simulink model "VLC"  (R2018b)
settings: Solver=FixedStepDiscrete  StartTime=0.0  StopTime=inf  FixedStep=0.01  RelTol=1e-3
PostLoadFcn:
  | if any(exist('dsrtsu_mdlpostloadfcn', 'file') ~= 0), dsrtsu_mdlpostloadfcn('Execute', bdroot); end
values from neighbouring files (symbols this model uses):
  m_Vehicle = 2000.0    [VLC_Local.sldd]
  P_A = 2.0    [VLC_Local.sldd]
  P_aDiffaF = 0.05    [VLC_Local.sldd]
  P_Cd = 0.29    [VLC_Local.sldd]
  P_Cf = 0.1    [VLC_Local.sldd]
  P_dAxMax = 2.0    [VLC_Local.sldd]
  P_dAxMin = -4.0    [VLC_Local.sldd]
  P_DC2ECMargin = 0.1    [VLC_Local.sldd]
  P_Dev4IEnd = 0.1    [VLC_Local.sldd]
  P_dIRamp = 1.0    [VLC_Local.sldd]
  P_DriveOffAdd = 400.0    [VLC_Local.sldd]
  P_dSlopeLim = 0.3    [VLC_Local.sldd]
  P_Ki = 0.08    [VLC_Local.sldd]
  P_Kp = 0.2    [VLC_Local.sldd]
  P_SlopeMax = 2.0    [VLC_Local.sldd]
  P_SlopeMin = 0.2    [VLC_Local.sldd]
  P_StandStillFactEC = 1.0    [VLC_Local.sldd]
  P_StsdCase = 1.0    [VLC_Local.sldd]
  P_StsddAxRamp = 1.0    [VLC_Local.sldd]
  P_tARefFilter = 0.2    [VLC_Local.sldd]
  P_tDriveOffThr = 5.0    [VLC_Local.sldd]
  P_tFxMergeFilter = 0.1    [VLC_Local.sldd]
  P_tSlopeFilter1 = 0.4    [VLC_Local.sldd]
  P_tSlopeFilter2 = 0.1    [VLC_Local.sldd]
  P_vDriveOffThr = 1.4    [VLC_Local.sldd]
  P_vLowSpd = 0.83    [VLC_Local.sldd]
  r_Wheel = 0.347    [VLC_Local.sldd]
  TransRatio = 7.38    [VLC_Local.sldd]
libraries: LPFilter x4
settings Model: DSRTSU_INTERNAL_RTI_VER=540  DSRTSU_INTERNAL_RTI_TYPE=rti1401  RTICANMMDATA=struct('GeneralSetupData',struct('modelroot','F:\DatabaseZO\08.Code\Model\ZOP_Integration','generalsettings',struct('filesettings',struct('destfolder',struct('Name','RTICANMM_FILES','Check',1),'buildfolder',struct('Name','.','Check',1),'AbsDestfolder',struct('Name','F:\DatabaseZO\08.Code\Model\ZOP_Integration\RTICANMM_FILES'),'AbsBuildfolder',struct('Name','F:\DatabaseZO\08.Code\Model\ZOP_Integration'))),'options',struct('addpaths',1,'rmpaths',1,'addtrcexclusion',logical(1),'cannavigator',struct('checkmonitoring',0),'show_usrtrc',0,'use_usrtrc',0),'advanced',struct('options',ones(1,100)),'MPSetup',{{}},'RTI',struct('Type','RTI1401','Ver','7.12','Date','02-May-2019'),'modelname','VLC','block','VLC'))  DSRTSU_INTERNAL_RTIFPGA=130  Creator=Administrator  LastModifiedBy=zjw
settings OptimizationCC: BlockReduction=off  ConditionallyExecuteInputs=off  OptimizeBlockIOStorage=off  BufferReuse=off  GlobalBufferReuse=off  ExpressionFolding=off  PassReuseOutputArgsThreshold=0  LocalBlockOutputs=off  OptimizeBlockOrder=speed  OptimizeDataStoreBuffers=off  BusAssignmentInplaceUpdate=off
settings DebuggingCC: ParameterTunabilityLossMsg=error  BusObjectLabelMismatch=none
settings HardwareCC: ProdBitPerPointer=32  ProdBitPerSizeT=32  ProdBitPerPtrDiffT=32  ProdLargestAtomicInteger=Integer  ProdEndianess=BigEndian  ProdWordSize=32  ProdHWDeviceType=Custom Processor->Custom  TargetIntDivRoundTo=Zero  TargetEndianess=BigEndian  TargetHWDeviceType=Custom Processor->Custom
settings ModelReferenceCC: ModelReferenceNumInstancesAllowed=Single
settings SFSimCC: MATLABDynamicMemAlloc=off
settings RTWCC: SystemTargetFile=rti1401.tlc  MakeCommand=make_rti  TemplateMakefile=rti1401.tmf  Description=dSPACE DS1401 Hardware Platform  GenerateReport=on  LaunchReport=on
settings CodeAppCC: OperatorAnnotations=on
settings STFCustomTargetCC: ParMdlRefBuildCompliant=on  SystemTargetFile=rti1401.tlc
settings GRTTargetCC: TargetLangStandard=C89/C90 (ANSI)  CompOptLevelCompliant=off  ConcurrentExecutionCompliant=off  CombineOutputUpdateFcns=off  MatFileLogging=off  CPPClassGenCompliant=off  UseToolchainInfoCompliant=off

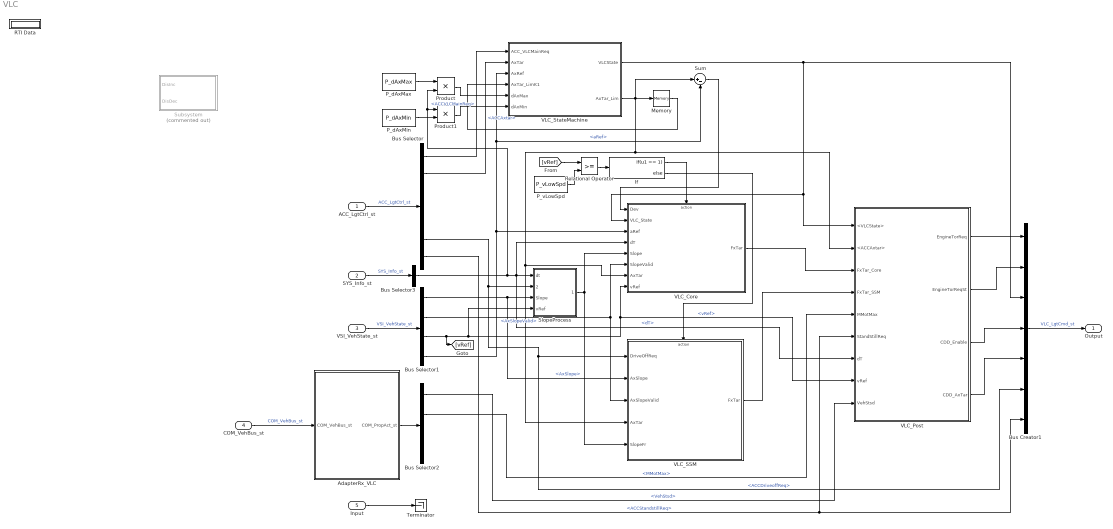
== system VLC ==
  ACC_LgtCtrl_st : Inport  OutDataTypeStr=Bus: ACC_LGTCTRL_ST  BusOutputAsStruct=on
  SYS_Info_st : Inport  Port=2  OutDataTypeStr=Bus: SYS_INFO_ST  BusOutputAsStruct=on
  VSI_VehState_st : Inport  Port=3  OutDataTypeStr=Bus: VSI_VEHSTATE_ST  BusOutputAsStruct=on
  COM_VehBus_st : Inport  Port=4  OutDataTypeStr=Bus: COM_VEHBUS_ST  BusOutputAsStruct=on
  Input : Inport  Port=5  OutDataTypeStr=Bus: COM_PROPACT_ST  BusOutputAsStruct=on
  AdapterRx_VLC : Subsystem
  Bus Creator1 : BusCreator  Inputs=7  OutDataTypeStr=Bus: VLC_LGTCMD_ST  NonVirtualBus=on
  Bus Selector : BusSelector  OutputSignals=ACCVLCMainReq,ACCAxtar,ACCAxTarUpperComfBand,ACCAxTarLowerComfBand,ACCBrkPrfrd,ACCDriveoffReq,ACCStandstillReq
  Bus Selector1 : BusSelector  OutputSignals=AxSlope,AxSlopeValid,vRef,aRef
  Bus Selector2 : BusSelector  OutputSignals=VehStsd,MMotMax,MMotMin,BrakeForce
  Bus Selector3 : BusSelector  OutputSignals=dT
  If : If  IfExpression=u1 == 1
  Memory : Memory
  P_dAxMax : Constant  Value=P_dAxMax
  P_dAxMin : Constant  Value=P_dAxMin
  P_vLowSpd : Constant  Value=P_vLowSpd
  Product : Product
  Product1 : Product
  RTI Data : Subsystem  Tag=struct('RTIDataServer',struct('RTIDataServerVs','2','RTIModelDescription','struct(''main'',''VLC'',''sub'','''',''isMp'',0)'))  LoadFcn="if exist('rtidc'), try,  rtidc('DataHostBlockClbLoad', gcbh); catch, disp(['Warning: ''LoadFcn'' for RTI Data block failed: ' lasterr]); end, end,"  mask(RTI_DATA_HOST){}
      mask help:
      | RTI Data Block.
      | This block is used by RTI to store internal model-dependent data.
      | Please keep this block on the root level of the model. Deleting this block will result in data loss.
      |
      | NEVER DELETE OR COPY THIS BLOCK!
      settings: CopyFcn="if exist('rtidc'), try,  rtidc('DataHostBlockClbCopy', gcbh); catch, disp(['Warning: ''CopyFcn'' for RTI Data block failed: ' lasterr]); end, end,"  DeleteFcn="if exist('rtidc'), try,  rtidc('DataHostBlockClbDelete', gcbh); catch, disp(['Warning: ''DeleteFcn'' for RTI Data block failed: ' lasterr]); end, end,"  ModelCloseFcn="if exist('rtidc'), try,  rtidc('DataHostBlockClbModelClose', gcbh); catch, disp(['Warning: ''ModelCloseFcn'' for RTI Data block failed: ' lasterr]); end, end,"  PreSaveFcn="if exist('rtidc'), try,  rtidc('DataHostBlockClbPreSave', gcbh); catch, disp(['Warning: ''PreSaveFcn'' for RTI Data block failed: ' lasterr]); end, end,"  PostSaveFcn="if exist('rtidc'), try,  rtidc('DataHostBlockClbPostSave', gcbh); catch, disp(['Warning: ''PostSaveFcn'' for RTI Data block failed: ' lasterr]); end, end,"  NameChangeFcn="if exist('rtidc'), try,  rtidc('DataHostBlockClbNameChange', gcbh); catch, disp(['Warning: ''NameChangeFcn'' for RTI Data block failed: ' lasterr]); end, end,"
      mask Help:
      | RTI Data Block.
      | This block is used by RTI to store internal model-dependent data.
      | Please keep this block on the root level of the model. Deleting this block will result in data loss.
      | 
      | NEVER DELETE OR COPY THIS BLOCK!
      mask Display:
      | text(0.5, 0.5, 'RTI Data', 'HorizontalAlignment', 'center');
      | plot([1 0]);
  Relational Operator : RelationalOperator  OutDataTypeStr=boolean  RndMeth=Simplest
  SlopeProcess : Subsystem
  Subsystem : Subsystem  Commented=on
  Sum : Sum  Inputs=|+-
  Terminator : Terminator
  VLC_Core : Subsystem
  VLC_Post : Subsystem
  VLC_SSM : Subsystem
  VLC_StateMachine : Stateflow chart  TreatAsAtomicUnit=on
  Output : Outport  OutDataTypeStr=Bus: VLC_LGTCMD_ST  BusOutputAsStruct=on
  wires:
  VSI_VehState_st/1 -> Bus Selector1/1  "VSI_VehState_st"
  If/1 -> VLC_Core/Action
  Bus Selector/2 -> VLC_StateMachine/2(AxTar)  "<ACCAxtar>"
  Bus Selector1/4 -> Sum/2, VLC_StateMachine/3(AxRef), VLC_Core/3(aRef)  "<aRef>"
  Bus Selector1/3 -> [vRef], SlopeProcess/4(vRef), VLC_Post/8(vRef), VLC_Core/8(vRef)  "<vRef>"
  If/2 -> VLC_SSM/Action
  Bus Selector/6 -> SlopeProcess/2(DriveOffReq), Bus Creator1/6, VLC_SSM/1(DriveOffReq)  "<ACCDriveoffReq>"
  Bus Selector1/2 -> VLC_SSM/3(AxSlopeValid), VLC_Core/6(SlopeValid)  "<AxSlopeValid>"
  Sum/1 -> VLC_Core/1(Dev)
  VLC_Core/1(FxTar) -> VLC_Post/3(FxTar_Core)
  VLC_SSM/1(FxTar) -> VLC_Post/4(FxTar_SSM)
  Bus Selector2/2 -> VLC_Post/5(MMotMax)  "<MMotMax>"
  Bus Selector/1 -> VLC_StateMachine/1(ACC_VLCMainReq)  "<ACCVLCMainReq>"
  VLC_StateMachine/1(VLCState) -> Bus Creator1/3, VLC_Post/1(<VLCState>), VLC_Core/2(VLC_State)
  VLC_StateMachine/2(AxTar_Lim) -> Memory/1, VLC_Post/2(<ACCAxtar>), VLC_SSM/4(AxTar), VLC_Core/7(AxTar), Sum/1
  Memory/1 -> VLC_StateMachine/4(AxTar_LimK1)
  VLC_Post/1(EngineTorReq) -> Bus Creator1/1
  VLC_Post/2(EngineTorReqSt) -> Bus Creator1/2
  VLC_Post/3(CDD_Enable) -> Bus Creator1/4
  VLC_Post/4(CDD_AxTar) -> Bus Creator1/5
  Bus Selector/7 -> Bus Creator1/7, VLC_Post/6(StandStillReq)  "<ACCStandstillReq>"
  SYS_Info_st/1 -> Bus Selector3/1  "SYS_Info_st"
  Bus Selector3/1 -> VLC_Post/7(dT), SlopeProcess/1(dt), VLC_Core/4(dT), Product/2, Product1/1  "<dT>"
  ACC_LgtCtrl_st/1 -> Bus Selector/1  "ACC_LgtCtrl_st"
  Product/1 -> VLC_StateMachine/5(dAxMax)
  P_dAxMax/1 -> Product/1
  AdapterRx_VLC/1(COM_PropAct_st) -> Bus Selector2/1
  COM_VehBus_st/1 -> AdapterRx_VLC/1(COM_VehBus_st)  "COM_VehBus_st"
  Bus Creator1/1 -> Output/1  "VLC_LgtCmd_st"
  Input/1 -> Terminator/1
  Bus Selector1/1 -> VLC_SSM/2(AxSlope), SlopeProcess/3(Slope)  "<AxSlope>"
  P_dAxMin/1 -> Product1/2
  Product1/1 -> VLC_StateMachine/6(dAxMin)
  SlopeProcess/1(SlopeFr) -> VLC_SSM/5(SlopeFr), VLC_Core/5(Slope)
  Bus Selector2/1 -> VLC_Post/9(VehStsd)  "<VehStsd>"
  P_vLowSpd/1 -> Relational Operator/2
  [vRef] -> Relational Operator/1
  Relational Operator/1 -> If/1

== system VLC/AdapterRx_VLC ==
  COM_VehBus_st : Inport  OutDataTypeStr=Bus: COM_VEHBUS_ST
  Bus Creator2 : BusCreator  Inputs=4  OutDataTypeStr=Bus: COM_PROPACT_ST  NonVirtualBus=on
  Bus Selector : BusSelector  OutputSignals=x251.VehSdslSts,xAC.EPTTrInptShaftMaxAvlblToq,xAC.EPTTrInptShaftMinAvlblToq,x24C.WhlBrkPrsSts
  Cast To Boolean : DataTypeConversion  OutDataTypeStr=single
  Divide : Product  Inputs=**
  Divide1 : Product  Inputs=**
  Logical Operator7 : Logic  Operator=NOT  AllPortsSameDT=off  OutDataTypeStr=boolean
  TransRatio : Constant  Value=TransRatio
  COM_PropAct_st : Outport  OutDataTypeStr=Bus: COM_PROPACT_ST
  wires:
  Bus Creator2/1 -> COM_PropAct_st/1  "COM_PropAct_st"
  Logical Operator7/1 -> Bus Creator2/4  "BrakeForce"
  Divide1/1 -> Bus Creator2/3  "MMotMin"
  Divide/1 -> Bus Creator2/2  "MMotMax"
  COM_VehBus_st/1 -> Bus Selector/1  "COM_VehBus_st"
  Bus Selector/4 -> Logical Operator7/1  "<WhlBrkPrsSts>"
  TransRatio/1 -> Divide/2, Divide1/2
  Bus Selector/2 -> Divide/1  "<EPTTrInptShaftMaxAvlblToq>"
  Bus Selector/3 -> Divide1/1  "<EPTTrInptShaftMinAvlblToq>"
  Bus Selector/1 -> Cast To Boolean/1  "<VehSdslSts>"
  Cast To Boolean/1 -> Bus Creator2/1  "VehStsd"

== system VLC/RTI Data ==
  RTI Data Store : Subsystem  Tag="struct('private',struct('version',struct('dsVer',uint32(2),'dsVerCreation',uint32(2),'RTI',struct('ver','7.12','type','RTI1401')),'access',struct('type','Model','isPerm',1,'created',['20-Nov-2020 12:07:07'],'modified',['07-Jan-2021 20:10:10'],'location','')),'public',struct('main',struct('data',[]),'sub',struct('name',{{'VLC'}},'data',{{struct('TH',struct('thTaskInfo',struct('taskType',{'TIMER','HWINT','TMRINT','SWINT','GLINT'},'tasksNumOf',{1,0,0,0,0},'srcIds',{{'TIMERA'},{},{},{},{}},'taskNames',{{['Timer Task 1']},{},{},{},{}})),'th_tc',struct('dataType','TASK','taskGroupId','','taskGroupList',{{}},'taskSchedulingPolicy','FCFS','taskType','TIMER','blkh',-1,'srcId','TIMERA','srcSgnName',['Timer A interrupt'],'srcCpuName','','taskName',['Timer Task 1  [0.01] s'],'taskNameDisplayExt','','smplTime',0.01,'smplTimeOffs',0,'hasFixedPriority',0,'priority',1,'hasFixedOvc',0,'ovcType',1,'ovcMax',1),'tc_th',struct('dataType','TASK','taskGroupId','','taskGroupList',{{}},'taskSchedulingPolicy','FCFS','taskType','TIMER','blkh',-1,'srcId','TIMERA','srcSgnName',['Timer A interrupt'],'srcCpuName','','taskName',['Timer Task 1  [0.01] s'],'taskNameDisplayExt','','smplTime',0.01,'smplTimeOffs',0,'hasFixedPriority',0,'priority',1,'hasFixedOvc',0,'ovcType',3,'ovcMax',1))}})))"  mask(RTI_DATA_STORE){}
      mask help:
      | RTI Data Store Block. This block is used by RTI to store internal model dependent data. Deleting this block will result in data loss.
      |
      | NEVER DELETE, COPY, OR MODIFY THIS BLOCK!
      mask Help:
      | RTI Data Store Block. This block is used by RTI to store internal model dependent data. Deleting this block will result in data loss.
      | 
      | NEVER DELETE, COPY, OR MODIFY THIS BLOCK!
      mask Display: text(0.5, 0.5, ' ', 'HorizontalAlignment', 'center');

== system VLC/SlopeProcess ==
  dt : Inport
  DriveOffReq : Inport  Port=2
  Slope : Inport  Port=3
  vRef : Inport  Port=4
  SlopeF : Subsystem
  SlopeFreeze : Subsystem
  SlopeFr : Outport
  wires:
  dt/1 -> SlopeFreeze/3(dT), SlopeF/1(dt)
  SlopeF/1(SlopeF) -> SlopeFreeze/4(SlopeF)
  SlopeFreeze/1(SlopeFreeze) -> SlopeFr/1
  Slope/1 -> SlopeF/2(Slope)
  vRef/1 -> SlopeFreeze/1(vVeh)
  DriveOffReq/1 -> SlopeFreeze/2(DriveOffReq)

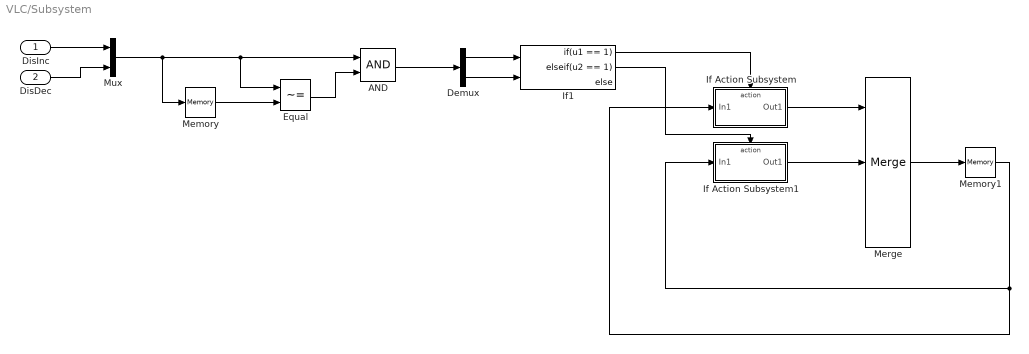
== system VLC/Subsystem ==
  DisInc : Inport
  DisDec : Inport  Port=2
  AND : Logic  AllPortsSameDT=off  OutDataTypeStr=boolean
  Demux : Demux  Outputs=2
  Equal : RelationalOperator  Operator=~=  OutDataTypeStr=boolean  RndMeth=Simplest
  If Action Subsystem : Subsystem  TreatAsAtomicUnit=on
  If Action Subsystem1 : Subsystem  TreatAsAtomicUnit=on
  If1 : If  NumInputs=2  IfExpression=u1 == 1  ElseIfExpressions=u2 == 1
  Memory : Memory
  Memory1 : Memory
  Merge : Merge  Inputs=3
  Mux : Mux  Inputs=2
  wires:
  Mux/1 -> Memory/1, Equal/1, AND/1
  Equal/1 -> AND/2
  Memory/1 -> Equal/2
  DisInc/1 -> Mux/1
  DisDec/1 -> Mux/2
  AND/1 -> Demux/1
  Demux/1 -> If1/1
  Demux/2 -> If1/2
  If1/1 -> If Action Subsystem/Action
  If Action Subsystem/1(Out1) -> Merge/1
  Merge/1 -> Memory1/1
  Memory1/1 -> If Action Subsystem1/1(In1), If Action Subsystem/1(In1)
  If Action Subsystem1/1(Out1) -> Merge/2
  If1/2 -> If Action Subsystem1/Action

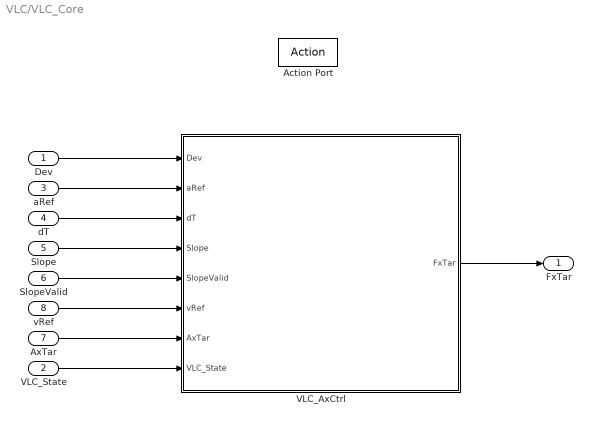
== system VLC/VLC_Core ==
  Dev : Inport
  VLC_State : Inport  Port=2
  aRef : Inport  Port=3
  dT : Inport  Port=4
  Slope : Inport  Port=5
  SlopeValid : Inport  Port=6
  AxTar : Inport  Port=7
  vRef : Inport  Port=8
  Action Port : ActionPort  ActionType=then
  VLC_AxCtrl : Subsystem
  FxTar : Outport
  wires:
  Dev/1 -> VLC_AxCtrl/1(Dev)
  VLC_AxCtrl/1(FxTar) -> FxTar/1
  aRef/1 -> VLC_AxCtrl/2(aRef)
  dT/1 -> VLC_AxCtrl/3(dT)
  Slope/1 -> VLC_AxCtrl/4(Slope)
  SlopeValid/1 -> VLC_AxCtrl/5(SlopeValid)
  vRef/1 -> VLC_AxCtrl/6(vRef)
  AxTar/1 -> VLC_AxCtrl/7(AxTar)
  VLC_State/1 -> VLC_AxCtrl/8(VLC_State)

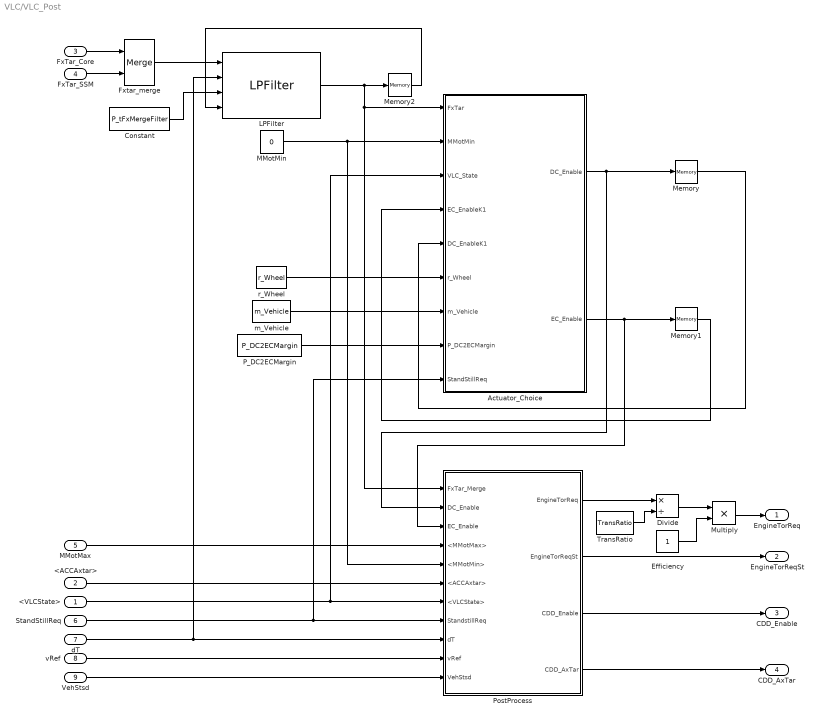
== system VLC/VLC_Post ==
  <VLCState> : Inport
  <ACCAxtar> : Inport  Port=2
  FxTar_Core : Inport  Port=3
  FxTar_SSM : Inport  Port=4
  MMotMax : Inport  Port=5
  StandStillReq : Inport  Port=6
  dT : Inport  Port=7
  vRef : Inport  Port=8
  VehStsd : Inport  Port=9
  Actuator_Choice : MATLAB Function  TreatAsAtomicUnit=on
  Constant : Constant  Value=P_tFxMergeFilter  OutDataTypeStr=single
  Divide : Product  Inputs=*/
  Efficiency : Constant
  Fxtar_merge : Merge
  LPFilter : LPFilter/LPFilter  SystemSampleTime=-1
      settings: SourceProductName=CustomLib
  MMotMin : Constant  Value=0  OutDataTypeStr=single
  Memory : Memory
  Memory1 : Memory
  Memory2 : Memory
  Multiply : Product  OutDataTypeStr=single
  P_DC2ECMargin : Constant  Value=P_DC2ECMargin
  PostProcess : Subsystem
  TransRatio : Constant  Value=TransRatio
  m_Vehicle : Constant  Value=m_Vehicle
  r_Wheel : Constant  Value=r_Wheel
  EngineTorReq : Outport
  EngineTorReqSt : Outport  Port=2
  CDD_Enable : Outport  Port=3
  CDD_AxTar : Outport  Port=4
  wires:
  MMotMin/1 -> Actuator_Choice/2(MMotMin), PostProcess/5(<MMotMin>)
  Actuator_Choice/1(DC_Enable) -> PostProcess/2(DC_Enable), Memory/1
  Memory/1 -> Actuator_Choice/5(DC_EnableK1)
  Actuator_Choice/2(EC_Enable) -> PostProcess/3(EC_Enable), Memory1/1
  Memory1/1 -> Actuator_Choice/4(EC_EnableK1)
  FxTar_SSM/1 -> Fxtar_merge/2
  FxTar_Core/1 -> Fxtar_merge/1
  MMotMax/1 -> PostProcess/4(<MMotMax>)
  <ACCAxtar>/1 -> PostProcess/6(<ACCAxtar>)
  <VLCState>/1 -> PostProcess/7(<VLCState>), Actuator_Choice/3(VLC_State)
  PostProcess/2(EngineTorReqSt) -> EngineTorReqSt/1
  PostProcess/3(CDD_Enable) -> CDD_Enable/1
  PostProcess/4(CDD_AxTar) -> CDD_AxTar/1
  r_Wheel/1 -> Actuator_Choice/6(r_Wheel)
  P_DC2ECMargin/1 -> Actuator_Choice/8(P_DC2ECMargin)
  m_Vehicle/1 -> Actuator_Choice/7(m_Vehicle)
  StandStillReq/1 -> PostProcess/8(StandstillReq), Actuator_Choice/9(StandStillReq)
  PostProcess/1(EngineTorReq) -> Divide/1
  TransRatio/1 -> Divide/2
  Divide/1 -> Multiply/1
  Multiply/1 -> EngineTorReq/1
  Efficiency/1 -> Multiply/2
  dT/1 -> PostProcess/9(dT), LPFilter/2
  LPFilter/1 -> Memory2/1, PostProcess/1(FxTar_Merge), Actuator_Choice/1(FxTar)
  Fxtar_merge/1 -> LPFilter/1
  Memory2/1 -> LPFilter/4
  Constant/1 -> LPFilter/3
  vRef/1 -> PostProcess/10(vRef)
  VehStsd/1 -> PostProcess/11(VehStsd)

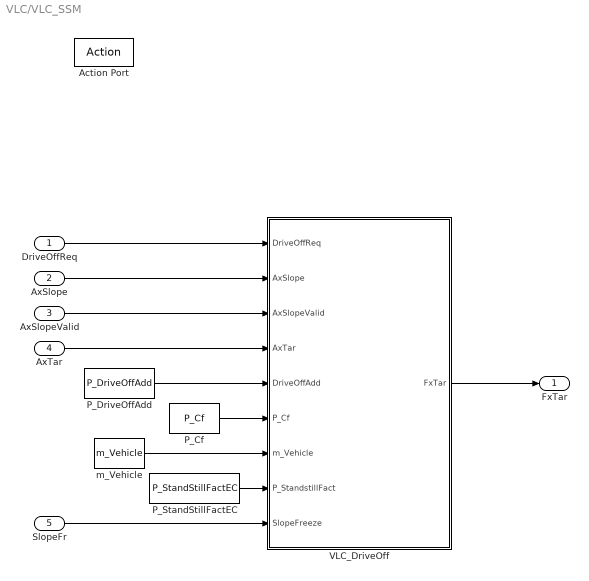
== system VLC/VLC_SSM ==
  DriveOffReq : Inport
  AxSlope : Inport  Port=2
  AxSlopeValid : Inport  Port=3
  AxTar : Inport  Port=4
  SlopeFr : Inport  Port=5
  Action Port : ActionPort  ActionType=else
  P_Cf : Constant  Value=P_Cf
  P_DriveOffAdd : Constant  Value=P_DriveOffAdd
  P_StandStillFactEC : Constant  Value=P_StandStillFactEC
  VLC_DriveOff : MATLAB Function  TreatAsAtomicUnit=on
  m_Vehicle : Constant  Value=m_Vehicle
  FxTar : Outport  OutDataTypeStr=single
  wires:
  DriveOffReq/1 -> VLC_DriveOff/1(DriveOffReq)
  AxSlope/1 -> VLC_DriveOff/2(AxSlope)
  VLC_DriveOff/1(FxTar) -> FxTar/1
  AxSlopeValid/1 -> VLC_DriveOff/3(AxSlopeValid)
  AxTar/1 -> VLC_DriveOff/4(AxTar)
  P_DriveOffAdd/1 -> VLC_DriveOff/5(DriveOffAdd)
  P_Cf/1 -> VLC_DriveOff/6(P_Cf)
  m_Vehicle/1 -> VLC_DriveOff/7(m_Vehicle)
  P_StandStillFactEC/1 -> VLC_DriveOff/8(P_StandstillFact)
  SlopeFr/1 -> VLC_DriveOff/9(SlopeFreeze)

== system VLC/RTI Data/RTI Data Store ==
  RTI Data Store : Subsystem  mask(RTI_DATA_STORE){}
      mask help:
      | RTI Data Store Block. This block is used by RTI to store internal model dependent data. Deleting this block will result in data loss.
      |
      | NEVER DELETE, COPY, OR MODIFY THIS BLOCK!
      mask Help:
      | RTI Data Store Block. This block is used by RTI to store internal model dependent data. Deleting this block will result in data loss.
      | 
      | NEVER DELETE, COPY, OR MODIFY THIS BLOCK!
      mask Display: text(0.5, 0.5, ' ', 'HorizontalAlignment', 'center');

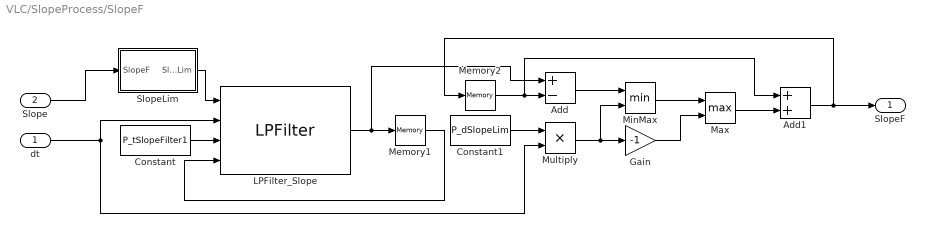
== system VLC/SlopeProcess/SlopeF ==
  dt : Inport
  Slope : Inport  Port=2
  Add : Sum  Inputs=+-
  Add1 : Sum
  Constant : Constant  Value=P_tSlopeFilter1  OutDataTypeStr=single
  Constant1 : Constant  Value=P_dSlopeLim  OutDataTypeStr=single
  Gain : Gain  Gain=-1
  LPFilter_Slope : LPFilter/LPFilter  SystemSampleTime=-1
      settings: SourceProductName=CustomLib
  Max : MinMax  Function=max  Inputs=2
  Memory1 : Memory
  Memory2 : Memory
  MinMax : MinMax  Inputs=2
  Multiply : Product
  SlopeLim : Subsystem
  SlopeF : Outport  OutDataTypeStr=single
  wires:
  Constant/1 -> LPFilter_Slope/3
  Gain/1 -> Max/2
  LPFilter_Slope/1 -> Add/1, Memory1/1
  Max/1 -> Add1/2
  Multiply/1 -> Gain/1, MinMax/2
  Add/1 -> MinMax/1
  Add1/1 -> SlopeF/1, Memory2/1
  Memory2/1 -> Add/2, Add1/1
  dt/1 -> Multiply/2, LPFilter_Slope/2
  MinMax/1 -> Max/1
  Constant1/1 -> Multiply/1
  Memory1/1 -> LPFilter_Slope/4
  SlopeLim/1(SlopeLim) -> LPFilter_Slope/1
  Slope/1 -> SlopeLim/1(SlopeF)

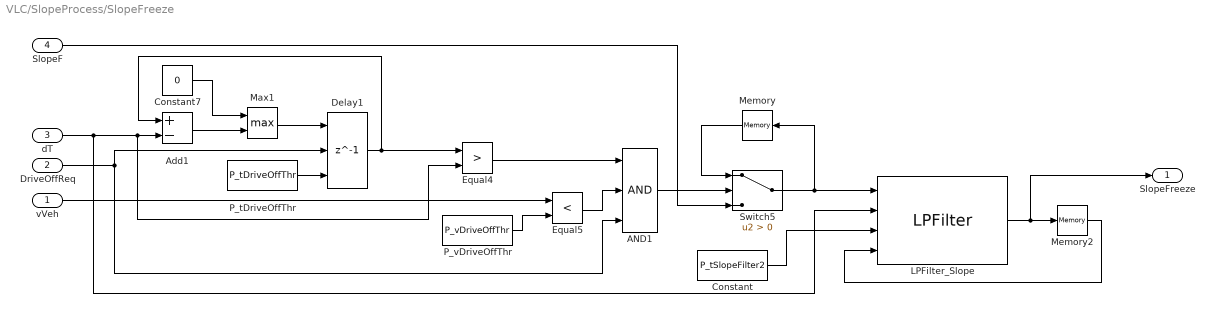
== system VLC/SlopeProcess/SlopeFreeze ==
  vVeh : Inport
  DriveOffReq : Inport  Port=2
  dT : Inport  Port=3
  SlopeF : Inport  Port=4
  AND1 : Logic  Inputs=3  AllPortsSameDT=off  OutDataTypeStr=boolean
  Add1 : Sum  Inputs=+-
  Constant : Constant  Value=P_tSlopeFilter2  OutDataTypeStr=single
  Constant7 : Constant  Value=0  OutDataTypeStr=single
  Delay1 : Delay  DelayLength=1  InitialConditionSource=Input port  ExternalReset=Rising
      settings: InputPortMap=u0,r5,p4
  Equal4 : RelationalOperator  Operator=>  OutDataTypeStr=boolean  RndMeth=Simplest
  Equal5 : RelationalOperator  Operator=<  OutDataTypeStr=boolean  RndMeth=Simplest
  LPFilter_Slope : LPFilter/LPFilter  SystemSampleTime=-1
      settings: SourceProductName=CustomLib
  Max1 : MinMax  Function=max  Inputs=2
  Memory : Memory
  Memory2 : Memory
  P_tDriveOffThr : Constant  Value=P_tDriveOffThr  OutDataTypeStr=single
  P_vDriveOffThr : Constant  Value=P_vDriveOffThr  OutDataTypeStr=single
  Switch5 : Switch  Criteria=u2 > Threshold
  SlopeFreeze : Outport
  wires:
  dT/1 -> LPFilter_Slope/2, Equal4/2, Add1/2
  Constant/1 -> LPFilter_Slope/3
  DriveOffReq/1 -> Delay1/2, AND1/3
  Delay1/1 -> Equal4/1, Add1/1
  LPFilter_Slope/1 -> SlopeFreeze/1, Memory2/1
  Memory2/1 -> LPFilter_Slope/4
  Equal4/1 -> AND1/1
  SlopeF/1 -> Switch5/3
  Add1/1 -> Max1/2
  Max1/1 -> Delay1/1
  Switch5/1 -> LPFilter_Slope/1, Memory/1
  P_tDriveOffThr/1 -> Delay1/3
  vVeh/1 -> Equal5/1
  Constant7/1 -> Max1/1
  Equal5/1 -> AND1/2
  P_vDriveOffThr/1 -> Equal5/2
  AND1/1 -> Switch5/2
  Memory/1 -> Switch5/1

== system VLC/Subsystem/If Action Subsystem ==
  In1 : Inport
  Action Port : ActionPort  ActionType=then
  Add : Sum
  Constant : Constant  OutDataTypeStr=single
  Out1 : Outport
  wires:
  In1/1 -> Add/1
  Add/1 -> Out1/1
  Constant/1 -> Add/2

== system VLC/Subsystem/If Action Subsystem1 ==
  In1 : Inport
  Action Port : ActionPort  ActionType=elseif
  Add : Sum  Inputs=+-
  Constant : Constant  OutDataTypeStr=single
  Out1 : Outport
  wires:
  In1/1 -> Add/1
  Add/1 -> Out1/1
  Constant/1 -> Add/2

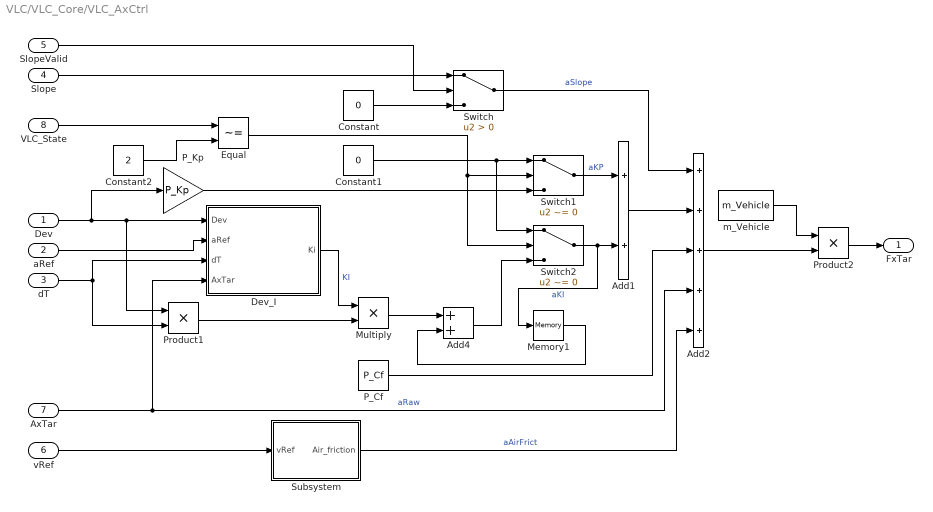
== system VLC/VLC_Core/VLC_AxCtrl ==
  Dev : Inport
  aRef : Inport  Port=2
  dT : Inport  Port=3
  Slope : Inport  Port=4
  SlopeValid : Inport  Port=5
  vRef : Inport  Port=6
  AxTar : Inport  Port=7
  VLC_State : Inport  Port=8
  Add1 : Sum
  Add2 : Sum  Inputs=+++++
  Add4 : Sum
  Constant : Constant  Value=0  OutDataTypeStr=single
  Constant1 : Constant  Value=0  OutDataTypeStr=single
  Constant2 : Constant  Value=2  OutDataTypeStr=single
  Dev_I : Subsystem
  Equal : RelationalOperator  Operator=~=  OutDataTypeStr=boolean  RndMeth=Simplest
  Memory1 : Memory
  Multiply : Product
  P_Cf : Constant  Value=P_Cf  OutDataTypeStr=single
  P_Kp : Gain  Gain=P_Kp
  Product1 : Product
  Product2 : Product
  Subsystem : Subsystem
  Switch : Switch  Criteria=u2 > Threshold
  Switch1 : Switch  Criteria=u2 ~= 0  Threshold=2
  Switch2 : Switch  Criteria=u2 ~= 0  Threshold=3
  m_Vehicle : Constant  Value=m_Vehicle
  FxTar : Outport
  wires:
  Dev/1 -> P_Kp/1, Product1/1, Dev_I/1(Dev)
  aRef/1 -> Dev_I/2(aRef)
  dT/1 -> Product1/2, Dev_I/3(dT)
  Constant/1 -> Switch/3
  Add2/1 -> Product2/2
  vRef/1 -> Subsystem/1(vRef)
  Product1/1 -> Multiply/2
  Memory1/1 -> Add4/2
  Product2/1 -> FxTar/1
  Switch1/1 -> Add1/1  "aKP"
  P_Kp/1 -> Switch1/3
  Constant1/1 -> Switch2/1, Switch1/1
  Add4/1 -> Switch2/3
  Slope/1 -> Switch/1
  Add1/1 -> Add2/2
  Switch/1 -> Add2/1  "aSlope"
  m_Vehicle/1 -> Product2/1
  P_Cf/1 -> Add2/3
  AxTar/1 -> Dev_I/4(AxTar), Add2/4  "aRaw"
  Subsystem/1(Air_friction) -> Add2/5  "aAirFrict"
  SlopeValid/1 -> Switch/2
  Dev_I/1(Ki) -> Multiply/1  "KI"
  Multiply/1 -> Add4/1
  VLC_State/1 -> Equal/1
  Constant2/1 -> Equal/2
  Equal/1 -> Switch2/2, Switch1/2
  Switch2/1 -> Add1/2, Memory1/1  "aKI"

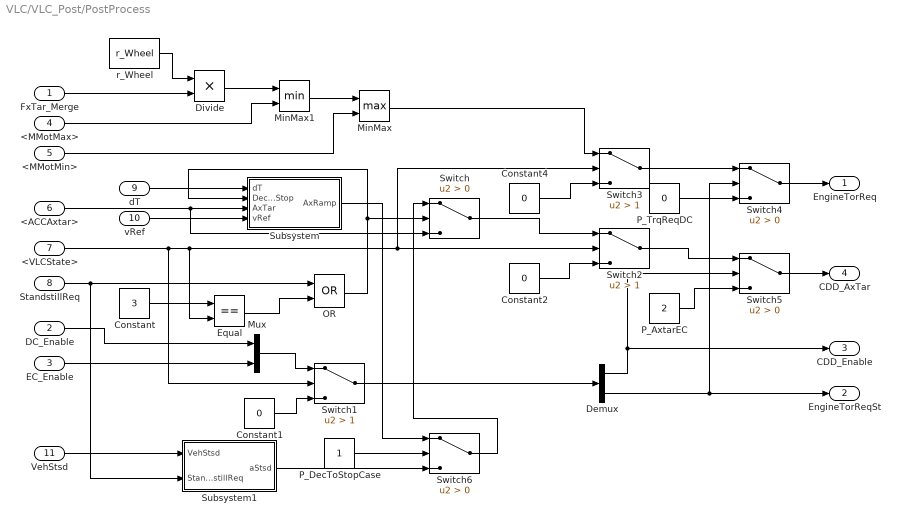
== system VLC/VLC_Post/PostProcess ==
  FxTar_Merge : Inport
  DC_Enable : Inport  Port=2
  EC_Enable : Inport  Port=3
  <MMotMax> : Inport  Port=4
  <MMotMin> : Inport  Port=5
  <ACCAxtar> : Inport  Port=6
  <VLCState> : Inport  Port=7
  StandstillReq : Inport  Port=8
  dT : Inport  Port=9
  vRef : Inport  Port=10
  VehStsd : Inport  Port=11
  Constant : Constant  Value=3
  Constant1 : Constant  Value=0
  Constant2 : Constant  Value=0
  Constant4 : Constant  Value=0
  Demux : Demux  Outputs=2
  Divide : Product  Inputs=**  OutDataTypeStr=single
  Equal : RelationalOperator  Operator===  OutDataTypeStr=boolean  RndMeth=Simplest
  MinMax : MinMax  Function=max  Inputs=2
  MinMax1 : MinMax  Inputs=2
  Mux : Mux  Inputs=2
  OR : Logic  Operator=OR  AllPortsSameDT=off  OutDataTypeStr=boolean
  P_AxtarEC : Constant  Value=2  OutDataTypeStr=single
  P_DecToStopCase : Constant  OutDataTypeStr=single
  P_TrqReqDC : Constant  Value=0  OutDataTypeStr=single
  Subsystem : Subsystem
  Subsystem1 : Subsystem
  Switch : Switch  Criteria=u2 > Threshold
  Switch1 : Switch  Criteria=u2 > Threshold  Threshold=1
  Switch2 : Switch  Criteria=u2 > Threshold  Threshold=1  OutDataTypeStr=single
  Switch3 : Switch  Criteria=u2 > Threshold  Threshold=1  OutDataTypeStr=single
  Switch4 : Switch  Criteria=u2 > Threshold  OutDataTypeStr=single
  Switch5 : Switch  Criteria=u2 > Threshold  OutDataTypeStr=single
  Switch6 : Switch  Criteria=u2 > Threshold
  r_Wheel : Constant  Value=r_Wheel
  EngineTorReq : Outport
  EngineTorReqSt : Outport  Port=2
  CDD_Enable : Outport  Port=3
  CDD_AxTar : Outport  Port=4
  wires:
  r_Wheel/1 -> Divide/1
  <VLCState>/1 -> Switch1/2, Switch2/2, Switch3/2, Equal/2
  DC_Enable/1 -> Mux/1
  Constant1/1 -> Switch1/3
  Demux/2 -> Switch4/2, EngineTorReqSt/1
  Mux/1 -> Switch1/1
  <MMotMax>/1 -> MinMax1/2
  <MMotMin>/1 -> MinMax/2
  Demux/1 -> Switch5/2, CDD_Enable/1
  MinMax1/1 -> MinMax/1
  Switch1/1 -> Demux/1
  Divide/1 -> MinMax1/1
  Constant2/1 -> Switch2/3
  EC_Enable/1 -> Mux/2
  FxTar_Merge/1 -> Divide/2
  MinMax/1 -> Switch3/1
  Constant4/1 -> Switch3/3
  Switch4/1 -> EngineTorReq/1
  Switch5/1 -> CDD_AxTar/1
  Switch3/1 -> Switch4/1
  Switch2/1 -> Switch5/1
  <ACCAxtar>/1 -> Switch/3, Subsystem/3(AxTar)
  Constant/1 -> Equal/1
  StandstillReq/1 -> Subsystem1/2(StandstillReq), OR/1
  OR/1 -> Subsystem/2(DecToStop), Switch/2
  Switch/1 -> Switch2/1
  dT/1 -> Subsystem/1(dT)
  Equal/1 -> OR/2
  vRef/1 -> Subsystem/4(vRef)
  P_AxtarEC/1 -> Switch5/3
  P_TrqReqDC/1 -> Switch4/3
  VehStsd/1 -> Subsystem1/1(VehStsd)
  Subsystem1/1(aStsd) -> Switch6/3
  P_DecToStopCase/1 -> Switch6/2
  Subsystem/1(AxRamp) -> Switch6/1
  Switch6/1 -> Switch/1

== system VLC/RTI Data/RTI Data Store/RTI Data Store ==
  RTI Data Store : Subsystem  mask(RTI_DATA_STORE){}
      mask help:
      | RTI Data Store Block. This block is used by RTI to store internal model dependent data. Deleting this block will result in data loss.
      |
      | NEVER DELETE, COPY, OR MODIFY THIS BLOCK!
      mask Help:
      | RTI Data Store Block. This block is used by RTI to store internal model dependent data. Deleting this block will result in data loss.
      | 
      | NEVER DELETE, COPY, OR MODIFY THIS BLOCK!
      mask Display: text(0.5, 0.5, ' ', 'HorizontalAlignment', 'center');

== system VLC/SlopeProcess/SlopeF/SlopeLim ==
  SlopeF : Inport
  Abs : Abs
  If : If  IfExpression=u1 == 1
  If Action Subsystem : Subsystem  TreatAsAtomicUnit=on
  If Action Subsystem1 : Subsystem  TreatAsAtomicUnit=on
  Merge : Merge
  P_SlopeMin : Constant  Value=P_SlopeMin  OutDataTypeStr=single
  Relational Operator : RelationalOperator  Operator=<=  OutDataTypeStr=boolean  RndMeth=Simplest
  SlopeLim : Outport
  wires:
  Relational Operator/1 -> If/1
  If Action Subsystem1/1(Out1) -> Merge/2
  Abs/1 -> Relational Operator/1
  If Action Subsystem/1(Out1) -> Merge/1
  Merge/1 -> SlopeLim/1
  If/1 -> If Action Subsystem/Action
  P_SlopeMin/1 -> Relational Operator/2
  SlopeF/1 -> If Action Subsystem1/1(In1), Abs/1
  If/2 -> If Action Subsystem1/Action

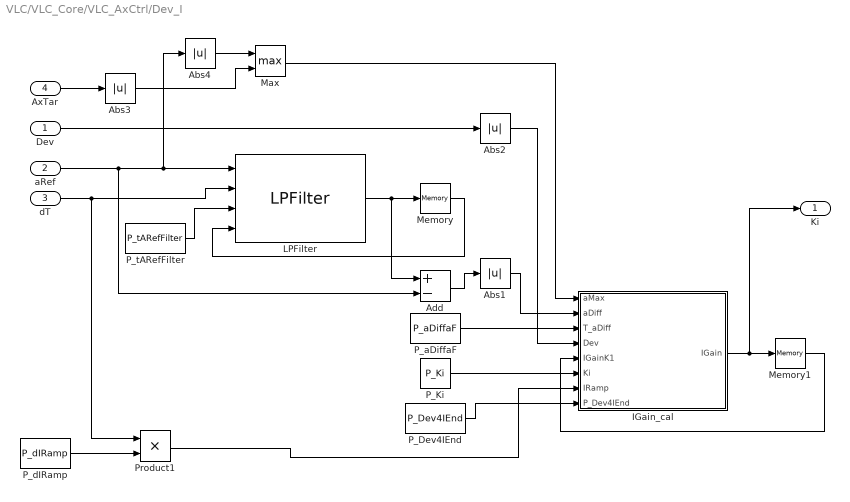
== system VLC/VLC_Core/VLC_AxCtrl/Dev_I ==
  Dev : Inport
  aRef : Inport  Port=2
  dT : Inport  Port=3
  AxTar : Inport  Port=4
  Abs{1..4} (4 alike) : Abs
  Add : Sum  Inputs=+-
  IGain_cal : MATLAB Function  TreatAsAtomicUnit=on
  LPFilter : LPFilter/LPFilter  SystemSampleTime=-1
      settings: SourceProductName=CustomLib
  Max : MinMax  Function=max  Inputs=2
  Memory : Memory
  Memory1 : Memory
  P_Dev4IEnd : Constant  Value=P_Dev4IEnd
  P_Ki : Constant  Value=P_Ki
  P_aDiffaF : Constant  Value=P_aDiffaF
  P_dIRamp : Constant  Value=P_dIRamp
  P_tARefFilter : Constant  Value=P_tARefFilter
  Product1 : Product
  Ki : Outport
  wires:
  Abs1/1 -> IGain_cal/2(aDiff)
  P_aDiffaF/1 -> IGain_cal/3(T_aDiff)
  IGain_cal/1(IGain) -> Ki/1, Memory1/1
  LPFilter/1 -> Memory/1, Add/1
  aRef/1 -> Abs4/1, LPFilter/1, Add/2
  Add/1 -> Abs1/1
  Memory/1 -> LPFilter/4
  P_tARefFilter/1 -> LPFilter/3
  dT/1 -> LPFilter/2, Product1/1
  P_Ki/1 -> IGain_cal/6(Ki)
  Dev/1 -> Abs2/1
  P_dIRamp/1 -> Product1/2
  Product1/1 -> IGain_cal/7(IRamp)
  P_Dev4IEnd/1 -> IGain_cal/8(P_Dev4IEnd)
  Memory1/1 -> IGain_cal/5(IGainK1)
  Abs2/1 -> IGain_cal/4(Dev)
  AxTar/1 -> Abs3/1
  Abs4/1 -> Max/1
  Abs3/1 -> Max/2
  Max/1 -> IGain_cal/1(aMax)

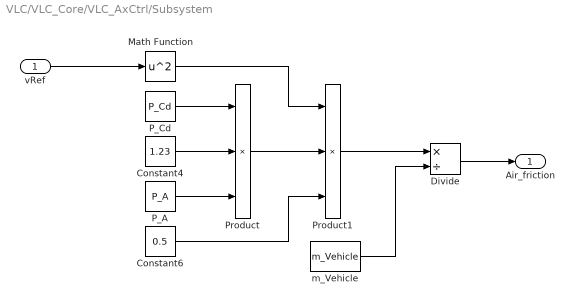
== system VLC/VLC_Core/VLC_AxCtrl/Subsystem ==
  vRef : Inport
  Constant4 : Constant  Value=1.23  OutDataTypeStr=single
  Constant6 : Constant  Value=0.5  OutDataTypeStr=single
  Divide : Product  Inputs=*/
  Math Function : Math  Operator=square  SaturateOnIntegerOverflow=on
  P_A : Constant  Value=P_A  OutDataTypeStr=single
  P_Cd : Constant  Value=P_Cd  OutDataTypeStr=single
  Product : Product  Inputs=3
  Product1 : Product  Inputs=3
  m_Vehicle : Constant  Value=m_Vehicle
  Air_friction : Outport
  wires:
  Constant4/1 -> Product/2
  P_A/1 -> Product/3
  Constant6/1 -> Product1/3
  vRef/1 -> Math Function/1
  P_Cd/1 -> Product/1
  Product/1 -> Product1/2
  Math Function/1 -> Product1/1
  Product1/1 -> Divide/1
  Divide/1 -> Air_friction/1
  m_Vehicle/1 -> Divide/2

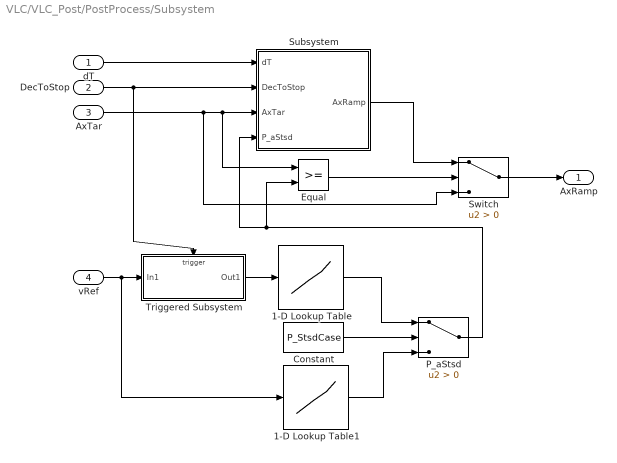
== system VLC/VLC_Post/PostProcess/Subsystem ==
  dT : Inport
  DecToStop : Inport  Port=2
  AxTar : Inport  Port=3
  vRef : Inport  Port=4
  1-D Lookup Table : Lookup_n-D  NumberOfTableDimensions=1  BreakpointsForDimension1=[1 3]  Table=[-1 -2]  ExtrapMethod=Clip  InternalRulePriority=Speed  RndMeth=Simplest  InputSameDT=on
  1-D Lookup Table1 : Lookup_n-D  NumberOfTableDimensions=1  BreakpointsForDimension1=[1 3]  Table=[-1 -2]  ExtrapMethod=Clip  InternalRulePriority=Speed  RndMeth=Simplest  InputSameDT=on
  Constant : Constant  Value=P_StsdCase  OutDataTypeStr=single
  Equal : RelationalOperator  OutDataTypeStr=boolean  RndMeth=Simplest
  P_aStsd : Switch  Criteria=u2 > Threshold
  Subsystem : Subsystem
  Switch : Switch  Criteria=u2 > Threshold
  Triggered Subsystem : Subsystem  TreatAsAtomicUnit=on
  AxRamp : Outport
  wires:
  dT/1 -> Subsystem/1(dT)
  DecToStop/1 -> Subsystem/2(DecToStop), Triggered Subsystem/Trigger
  AxTar/1 -> Subsystem/3(AxTar), Equal/1, Switch/3
  Switch/1 -> AxRamp/1
  Subsystem/1(AxRamp) -> Switch/1
  Equal/1 -> Switch/2
  P_aStsd/1 -> Subsystem/4(P_aStsd), Equal/2
  vRef/1 -> 1-D Lookup Table1/1, Triggered Subsystem/1(In1)
  Triggered Subsystem/1(Out1) -> 1-D Lookup Table/1
  Constant/1 -> P_aStsd/2
  1-D Lookup Table/1 -> P_aStsd/1
  1-D Lookup Table1/1 -> P_aStsd/3

== system VLC/VLC_Post/PostProcess/Subsystem1 ==
  VehStsd : Inport
  StandstillReq : Inport  Port=2
  AND : Logic  AllPortsSameDT=off  OutDataTypeStr=boolean
  Constant3 : Constant  OutDataTypeStr=single
  Equal1 : RelationalOperator  Operator===  OutDataTypeStr=boolean  RndMeth=Simplest
  Equal2 : RelationalOperator  Operator===  OutDataTypeStr=boolean  RndMeth=Simplest
  If : If  IfExpression=u1 == 1
  If Action Subsystem : Subsystem  TreatAsAtomicUnit=on
  If Action Subsystem1 : Subsystem  TreatAsAtomicUnit=on
  Merge : Merge
  aStsd : Outport
  wires:
  VehStsd/1 -> Equal1/1
  Constant3/1 -> Equal2/1, Equal1/2
  StandstillReq/1 -> Equal2/2
  Equal1/1 -> AND/1
  Equal2/1 -> AND/2
  AND/1 -> If/1
  If/1 -> If Action Subsystem/Action
  If/2 -> If Action Subsystem1/Action
  If Action Subsystem/1(Out1) -> Merge/1
  If Action Subsystem1/1(Out1) -> Merge/2
  Merge/1 -> aStsd/1

== system VLC/RTI Data/RTI Data Store/RTI Data Store/RTI Data Store ==
  RTI Data Store : Subsystem  mask(RTI_DATA_STORE){}
      mask help:
      | RTI Data Store Block. This block is used by RTI to store internal model dependent data. Deleting this block will result in data loss.
      |
      | NEVER DELETE, COPY, OR MODIFY THIS BLOCK!
      mask Help:
      | RTI Data Store Block. This block is used by RTI to store internal model dependent data. Deleting this block will result in data loss.
      | 
      | NEVER DELETE, COPY, OR MODIFY THIS BLOCK!
      mask Display: text(0.5, 0.5, ' ', 'HorizontalAlignment', 'center');

== system VLC/SlopeProcess/SlopeF/SlopeLim/If Action Subsystem ==
  Action Port : ActionPort  ActionType=then
  Constant : Constant  Value=0  OutDataTypeStr=single
  Out1 : Outport
  wires:
  Constant/1 -> Out1/1

== system VLC/SlopeProcess/SlopeF/SlopeLim/If Action Subsystem1 ==
  In1 : Inport
  Action Port : ActionPort  ActionType=else
  Gain : Gain  Gain=-1
  Max : MinMax  Inputs=2
  Min : MinMax  Function=max  Inputs=2
  P_SlopeMax : Constant  Value=P_SlopeMax  OutDataTypeStr=single
  Out1 : Outport
  wires:
  In1/1 -> Max/1
  P_SlopeMax/1 -> Max/2, Gain/1
  Min/1 -> Out1/1
  Max/1 -> Min/1
  Gain/1 -> Min/2

== system VLC/VLC_Post/PostProcess/Subsystem/Subsystem ==
  dT : Inport
  DecToStop : Inport  Port=2
  AxTar : Inport  Port=3
  P_aStsd : Inport  Port=4
  Add1 : Sum  Inputs=+-
  Delay1 : Delay  DelayLength=1  InitialConditionSource=Input port  ExternalReset=Rising
      settings: InputPortMap=u0,r5,p4
  Max : MinMax  Function=max  Inputs=2
  Multiply : Product
  P_StsddAxRamp : Constant  Value=P_StsddAxRamp  OutDataTypeStr=single
  AxRamp : Outport
  wires:
  Add1/1 -> Max/2
  DecToStop/1 -> Delay1/2
  P_StsddAxRamp/1 -> Multiply/1
  Delay1/1 -> AxRamp/1, Add1/1
  Multiply/1 -> Add1/2
  AxTar/1 -> Delay1/3
  dT/1 -> Multiply/2
  P_aStsd/1 -> Max/1
  Max/1 -> Delay1/1

== system VLC/VLC_Post/PostProcess/Subsystem/Triggered Subsystem ==
  In1 : Inport
  Trigger : TriggerPort  VariantControl=Variant
  Out1 : Outport
  wires:
  In1/1 -> Out1/1

== system VLC/VLC_Post/PostProcess/Subsystem1/If Action Subsystem ==
  Action Port : ActionPort  ActionType=then
  Constant : Constant  Value=-1  OutDataTypeStr=single
  Out1 : Outport
  wires:
  Constant/1 -> Out1/1

== system VLC/VLC_Post/PostProcess/Subsystem1/If Action Subsystem1 ==
  Action Port : ActionPort  ActionType=else
  P_aStsd : Constant  Value=-0.4  OutDataTypeStr=single
  Out1 : Outport
  wires:
  P_aStsd/1 -> Out1/1

== system VLC/RTI Data/RTI Data Store/RTI Data Store/RTI Data Store/RTI Data Store ==

== matlab function VLC/VLC_SSM/VLC_DriveOff ==
  data: DriveOffReq input; AxSlope input; AxSlopeValid input; AxTar input; DriveOffAdd input; FxTar output; P_Cf input; m_Vehicle input; P_StandstillFact input; SlopeFreeze input
function FxTar = fcn2(DriveOffReq,AxSlope,AxSlopeValid,AxTar,DriveOffAdd,P_Cf,m_Vehicle,P_StandstillFact,SlopeFreeze)

if (DriveOffReq)
    FxTar = m_Vehicle * (AxTar + SlopeFreeze*AxSlopeValid + P_Cf) + DriveOffAdd;
else
    FxTar = (P_StandstillFact * AxTar + AxSlope*AxSlopeValid + P_Cf) * m_Vehicle;
end

== matlab function VLC/VLC_Core/VLC_AxCtrl/Dev_I/IGain_cal ==
  data: aMax input; aDiff input; IGain output; T_aDiff input; Dev input; IGainK1 input single; Ki input; IRamp input; P_Dev4IEnd input
function IGain = IGain(aMax,aDiff,T_aDiff,Dev,IGainK1,Ki,IRamp,P_Dev4IEnd)

if (aDiff <= T_aDiff) && (Dev <= P_Dev4IEnd) && (aMax < 0.5) && (IGainK1 ~= Ki)
    IGain = Ki;
elseif (aDiff > T_aDiff) || (Dev > P_Dev4IEnd) || (aMax >= 0.5)
    IGain = IGainK1 - IRamp;
    IGain = max(IGain,0);
else
    IGain = IGainK1;
end

== stateflow chart VLC/VLC_StateMachine ==
  state OFF
    entry:
    VLCState = 0;
    AxTar_Lim = 0;
  state Standby
    entry:
    VLCState = 1;
    AxTar_Lim = 0;
  state Standstill
    entry:
    VLCState = 3;
    du:
    AxTar_Lim = max(min((AxTar - AxTar_LimK1), dAxMax), dAxMin) + AxTar_LimK1;
  state Suspend
    entry:
    VLCState = 4;
    du:
    AxTar_Lim = max(min((AxTar - AxTar_LimK1), dAxMax), dAxMin) + AxTar_LimK1;
  state Drive
    entry:
    VLCState = 2;
    AxTar_Lim = AxRef;
    du:
    AxTar_Lim = max(min((AxTar - AxTar_LimK1), dAxMax), dAxMin) + AxTar_LimK1;
  note: MainState
      | 0 OFF
      | 1 Standby
      | 2 Drive
      | 3 Standstill
      | 4 Suspend
  Suspend -> Standstill [order 4] : [ACC_VLCMainReq == 3]
  Standstill -> OFF [order 3] : [ACC_VLCMainReq == 0]
  (default) -> OFF
  OFF -> Standby : [ACC_VLCMainReq == 1]
  Standby -> Standstill [order 2] : [ACC_VLCMainReq == 3]
  Standstill -> Suspend [order 4] : [ACC_VLCMainReq == 4]
  Suspend -> Standby [order 2] : [ACC_VLCMainReq == 1]
  Standby -> OFF [order 3] : [ACC_VLCMainReq == 0]
  Standstill -> Standby [order 2] : [ACC_VLCMainReq == 1]
  Standby -> Drive [order 1] : [ACC_VLCMainReq == 2]
  Drive -> OFF [order 4] : [ACC_VLCMainReq == 0]
  Suspend -> OFF [order 3] : [ACC_VLCMainReq == 0]
  Drive -> Standby [order 3] : [ACC_VLCMainReq == 1]
  Drive -> Standstill [order 1] : [ACC_VLCMainReq == 3]
  Standstill -> Drive [order 1] : [ACC_VLCMainReq == 2]
  Suspend -> Drive [order 1] : [ACC_VLCMainReq == 2]
  Drive -> Suspend [order 2] : [ACC_VLCMainReq == 4]
  data: ACC_VLCMainReq input single; VLCState output single; AxTar input single; AxRef input single; AxTar_Lim output single; AxTar_LimK1 input single; dAxMax input single; dAxMin input single

== matlab function VLC/VLC_Post/Actuator_Choice ==
  data: FxTar input; DC_Enable output; MMotMin input; VLC_State input; EC_Enable output; EC_EnableK1 input; DC_EnableK1 input; r_Wheel input; m_Vehicle input; P_DC2ECMargin input; StandStillReq input
function [DC_Enable,EC_Enable] = fcn1(FxTar,MMotMin,VLC_State,EC_EnableK1,DC_EnableK1,r_Wheel,m_Vehicle,P_DC2ECMargin,StandStillReq)

if (VLC_State == 4)
    DC_Enable = 0;
    EC_Enable = 1;
elseif (StandStillReq||(VLC_State == 3))
    DC_Enable = 1;
    EC_Enable = 0;
elseif (FxTar < MMotMin/r_Wheel)
    DC_Enable = 1;
    EC_Enable = 0;
elseif ( FxTar > P_DC2ECMargin * m_Vehicle + MMotMin/r_Wheel)
    DC_Enable = 0;
    EC_Enable = 1;
else
    EC_Enable = EC_EnableK1;
    DC_Enable = DC_EnableK1;
end
